simulink model "half_bridge_llc_resonant_converter"  (R2019a)
settings: Solver=VariableStepAuto  StartTime=0.0  StopTime=0.005  RelTol=1e-3
libraries: powerlib x18
settings Model: Creator=Deepak  LastModifiedBy=Deepak

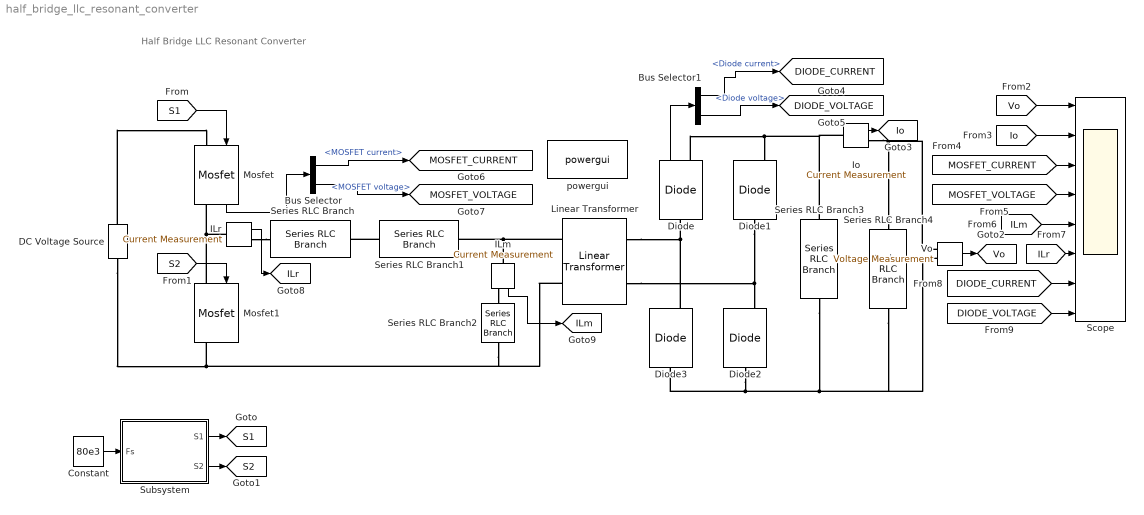
== system half_bridge_llc_resonant_converter ==
  note: Half Bridge LLC Resonant Converter
  Bus Selector : BusSelector  OutputSignals=MOSFET current,MOSFET voltage
  Bus Selector1 : BusSelector  OutputSignals=Diode current,Diode voltage
  Constant : Constant  Value=80e3
  DC Voltage Source : powerlib/Electrical Sources/DC Voltage Source  Amplitude=398  Measurements=None
      settings: SourceProductName=Simscape Electrical
  Diode{,1..3} (4 alike) : powerlib/Power Electronics/Diode  Ron=0.001  Lon=0  Vf=0.8  IC=0  UseSnubber=0  Rs=500  Cs=250e-9  Measurements=on
      settings: SourceProductName=Simscape Electrical
  ILm : powerlib/Measurements/Current Measurement  PhasorSimulation=off  OutputType=Complex  PSBequivalent=0
      settings: SourceProductName=Simscape Electrical
  ILr : powerlib/Measurements/Current Measurement  PhasorSimulation=off  OutputType=Complex  PSBequivalent=0
      settings: SourceProductName=Simscape Electrical
  Io : powerlib/Measurements/Current Measurement  PhasorSimulation=off  OutputType=Complex  PSBequivalent=0
      settings: SourceProductName=Simscape Electrical
  Linear Transformer : powerlib/Elements/Linear Transformer  UNITS=SI  NominalPower=[ 700 100e3 ]  winding1=[3.39 0 0]  winding2=[1 0 0]  ThreeWindings=off  winding3=[3.15e+05 0.7938 0.084225]  RmLm=[100 0]  Measurements=None  DataType=on
      settings: SourceProductName=Simscape Electrical
  Mosfet : powerlib/Power Electronics/Mosfet  Ron=0.1  Lon=0  Rd=0.01  Vfd=0  IC=0  Rs=1e5  Cs=inf  Measurements=on
      settings: SourceProductName=Simscape Electrical
  Mosfet1 : powerlib/Power Electronics/Mosfet  Ron=0.1  Lon=0  Rd=0.01  Vfd=0  IC=0  Rs=1e5  Cs=inf  Measurements=on
      settings: SourceProductName=Simscape Electrical
  Scope : Scope  NumInputPorts=8
  Series RLC Branch : powerlib/Elements/Series RLC Branch  LConnTagsString=__new0  RConnTagsString=__new0  BranchType=L  Resistance=1  Inductance=22.6e-6  SetiL0=off  InitialCurrent=0  Capacitance=1e-6  Setx0=off  InitialVoltage=0  Measurements=None
      settings: SourceProductName=Simscape Electrical
  Series RLC Branch1 : powerlib/Elements/Series RLC Branch  LConnTagsString=__new0  RConnTagsString=__new0  BranchType=C  Resistance=1  Inductance=1e-3  SetiL0=off  InitialCurrent=0  Capacitance=112e-9  Setx0=off  InitialVoltage=0  Measurements=None
      settings: SourceProductName=Simscape Electrical
  Series RLC Branch2 : powerlib/Elements/Series RLC Branch  LConnTagsString=__new0  RConnTagsString=__new0  BranchType=L  Resistance=1  Inductance=3.5*22.6e-6  SetiL0=off  InitialCurrent=0  Capacitance=1e-6  Setx0=off  InitialVoltage=0  Measurements=None
      settings: SourceProductName=Simscape Electrical
  Series RLC Branch3 : powerlib/Elements/Series RLC Branch  LConnTagsString=__new0  RConnTagsString=__new0  BranchType=C  Resistance=1  Inductance=1e-3  SetiL0=off  InitialCurrent=0  Capacitance=100e-6  Setx0=off  InitialVoltage=0  Measurements=None
      settings: SourceProductName=Simscape Electrical
  Series RLC Branch4 : powerlib/Elements/Series RLC Branch  LConnTagsString=__new0  RConnTagsString=__new0  BranchType=R  Resistance=4.833  Inductance=1e-3  SetiL0=off  InitialCurrent=0  Capacitance=1e-6  Setx0=off  InitialVoltage=0  Measurements=None
      settings: SourceProductName=Simscape Electrical
  Subsystem : Subsystem
  Vo : powerlib/Measurements/Voltage Measurement  PhasorSimulation=off  OutputType=Complex  PSBequivalent=0
      settings: SourceProductName=Simscape Electrical
  powergui : powerlib/powergui  Priority=1  SimulationMode=Continuous  SampleTime=50e-6  frequency=60  Iterations=50  frequencyindice=0  Pbase=100e6  ErrMax=1e-4  UnitsV=kV  UnitsW=MW  buscounter=0  FunctionMessages=off  echomessages=off  EnableUseOfTLC=off  CurrentSourceSwitches=off  DisableSnubberDevices=off  DisableRonSwitches=off  DisableVfSwitches=off  DisplayEquations=off  AutomaticDiscreteSolvers=off  SolverType=Tustin/Backward Euler (TBE)  Interpol=off  ExternalGateDelay=off  methode=off  Ts=100  x0status=blocks  SPID=on  SwTol=0  HookPort=off  NonlinearTolerance=0  nMaxIteration=15  ContinueOnMaxIteration=off  RestoreLinks=warning  ResistiveCurrentMeasurement=off  Frange=[0:2:500]  Ylog=off  Xlog=on  ShowGrid=off  save=off  variable=ZData  structure=0  ZoomFFT=off  StartTime=0.0  cycles=1  DisplayStyle=1  fundamental=60  FreqAxis=off  MaxFrequency=1000  frequencyindicesteady=1  RmsSteady=1  display=off
      settings: SourceProductName=Simscape Electrical
  tag scope: DIODE_CURRENT=global, DIODE_VOLTAGE=global, ILm=global, ILr=global, Io=global, MOSFET_CURRENT=global, MOSFET_VOLTAGE=global, S1=global, S2=global, Vo=global
  wires:
  Subsystem/1(S1) -> [S1]
  Subsystem/2(S2) -> [S2]
  [S1] -> Mosfet/1
  [S2] -> Mosfet1/1
  Mosfet/1 -> Bus Selector/1
  Diode/1 -> Bus Selector1/1
  Bus Selector1/1 -> [DIODE_CURRENT]  "<Diode current>"
  Constant/1 -> Subsystem/1(" Fs")
  Vo/1 -> [Vo]
  Io/1 -> [Io]
  Bus Selector1/2 -> [DIODE_VOLTAGE]  "<Diode voltage>"
  Bus Selector/1 -> [MOSFET_CURRENT]  "<MOSFET current>"
  Bus Selector/2 -> [MOSFET_VOLTAGE]  "<MOSFET voltage>"
  ILr/1 -> [ILr]
  ILm/1 -> [ILm]
  [Vo] -> Scope/1
  [Io] -> Scope/2
  [MOSFET_CURRENT] -> Scope/3
  [MOSFET_VOLTAGE] -> Scope/4
  [ILm] -> Scope/5
  [ILr] -> Scope/6
  [DIODE_CURRENT] -> Scope/7
  [DIODE_VOLTAGE] -> Scope/8
  connections:
  Mosfet1/LConn1 -- ILr/LConn1 -- Mosfet/RConn1
  DC Voltage Source/RConn1 -- Mosfet/LConn1
  DC Voltage Source/LConn1 -- Series RLC Branch2/RConn1 -- Linear Transformer/LConn2 -- Mosfet1/RConn1
  Series RLC Branch1/LConn1 -- Series RLC Branch/RConn1
  Linear Transformer/LConn1 -- Series RLC Branch1/RConn1 -- ILm/LConn1
  Diode3/RConn1 -- Linear Transformer/RConn1 -- Diode/LConn1
  Diode1/LConn1 -- Linear Transformer/RConn2 -- Diode2/RConn1
  Diode2/LConn1 -- Vo/LConn2 -- Series RLC Branch4/RConn1 -- Series RLC Branch3/RConn1 -- Diode3/LConn1
  Diode/RConn1 -- Series RLC Branch3/LConn1 -- Io/LConn1 -- Diode1/RConn1
  Io/RConn1 -- Vo/LConn1 -- Series RLC Branch4/LConn1
  ILr/RConn1 -- Series RLC Branch/LConn1
  ILm/RConn1 -- Series RLC Branch2/LConn1

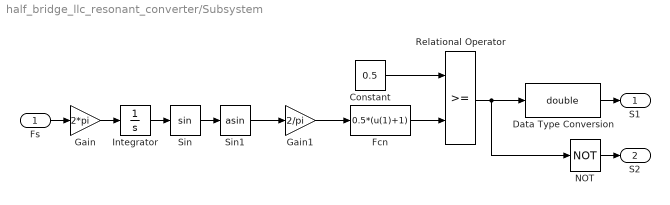
== system half_bridge_llc_resonant_converter/Subsystem ==
  " Fs" : Inport
  Constant : Constant  Value=0.5
  Data Type Conversion : DataTypeConversion  OutDataTypeStr=double
  Fcn : Fcn  Expr=0.5*(u(1)+1)
  Gain : Gain  Gain=2*pi
  Gain1 : Gain  Gain=2/pi
  Integrator : Integrator
  NOT : Logic  Operator=NOT  IconShape=distinctive  AllPortsSameDT=off  OutDataTypeStr=boolean
  Relational Operator : RelationalOperator  OutDataTypeStr=boolean  RndMeth=Simplest
  Sin : Trigonometry
  Sin1 : Trigonometry  Operator=asin
  S1 : Outport
  S2 : Outport  Port=2
  wires:
  Integrator/1 -> Sin/1
  Constant/1 -> Relational Operator/1
  Sin1/1 -> Gain1/1
  Sin/1 -> Sin1/1
  Relational Operator/1 -> NOT/1, Data Type Conversion/1
  Gain/1 -> Integrator/1
  Gain1/1 -> Fcn/1
  Fcn/1 -> Relational Operator/2
  NOT/1 -> S2/1
  " Fs"/1 -> Gain/1
  Data Type Conversion/1 -> S1/1
